simulink model "robocup_model"  (Simulink 8.6)
settings: Solver=ode45  StartTime=0.0  StopTime=8  RelTol=1e-3
libraries: fuzblock x3, simulink x3
settings Model: Creator=justbuchanan  LastModifiedBy=abdullah
settings SolverCC: ZeroCrossControl=EnableAll  ZeroCrossAlgorithm=Adaptive
settings DataIOCC: SignalLoggingSaveFormat=Dataset
settings OptimizationCC: BlockReduction=off  BufferReuse=off  ExpressionDepthLimit=128  SimCompilerOptimization=on
settings DebuggingCC: UnderspecifiedInitializationDetection=Simplified  MergeDetectMultiDrivingBlocksExec=error  FcnCallInpInsideContextMsg=EnableAllAsError  StateNameClashWarn=none
settings HardwareCC: ProdLargestAtomicInteger=Long  ProdLargestAtomicFloat=Double  ProdEndianess=LittleEndian  ProdHWDeviceType=ARM Compatible->ARM Cortex
settings GRTTargetCC: CombineOutputUpdateFcns=on  GRTInterface=off
settings ConfigComp: CovSFcnEnable=off

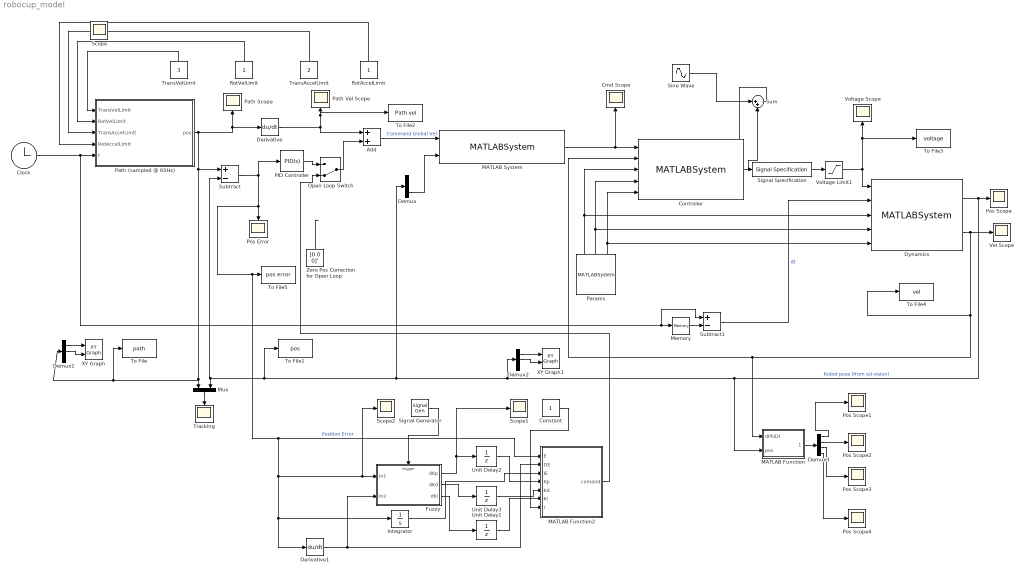
== system robocup_model ==
  Add : Sum
  Clock : Clock
  Cmd Scope : Scope
  Constant : Constant
  Controller : MATLABSystem  System=RobotLqr  trans_vel_weight=5  rot_vel_weight=0.1  u_weight=1  SimulateUsing=Interpreted execution
      mask Type: RobotLqr
      mask Display:
      | disp('RobotLqr');
      | port_label('input',1,'Cmd Velocity');
      | port_label('input',2,'Curr. Velocity');
      | port_label('input',3,'A_1');
      | port_label('input',4,'A_2');
      | port_label('input',5,'B');
      | port_label('output',1,'u');
  Demux : Demux  Outputs=3
  Demux1 : Demux  Outputs=3
  Demux2 : Demux  Outputs=3
  Demux3 : Demux
  Derivative : Derivative
  Derivative1 : Derivative
  Dynamics : MATLABSystem  System=Robot  SimulateUsing=Interpreted execution
      mask Type: Robot
      mask Display:
      | disp(['RoboCup Robot' char(10) 'Dynamics']);
      | port_label('input',1,'Motor Voltages');
      | port_label('input',2,'dt');
      | port_label('input',3,'A_1');
      | port_label('input',4,'A_2');
      | port_label('input',5,'B');
      | port_label('output',1,'Robot pose');
      | port_label('output',2,'Robot velocity');
  Fuzzy : Subsystem
  Integrator : Integrator
  MATLAB Function : MATLAB Function  TreatAsAtomicUnit=on
  MATLAB Function2 : MATLAB Function  TreatAsAtomicUnit=on
  MATLAB System : MATLABSystem  System=Global2Body  SimulateUsing=Code generation
      mask Type: Global2Body
      mask Display:
      | disp('Global2Body');
      | port_label('input',1,'Global Velocity');
      | port_label('input',2,'Robot angle');
      | port_label('output',1,'Body Velocity');
  Memory : Memory  X0=-0.1
  Mux : Mux  Inputs=2
  Open Loop Switch : ManualSwitch  CurrentSetting=0
  PID Controller : simulink/Continuous/PID Controller  Controller=PID  TimeDomain=Continuous-time  SampleTime=-1  IntegratorMethod=Forward Euler  FilterMethod=Forward Euler  Form=Parallel  UseFilter=on  ControllerParametersSource=internal  P=8  I=4  D=0  N=100  InitialConditionSource=internal  InitialConditionForIntegrator=0  InitialConditionForFilter=0  ExternalReset=none  LimitOutput=off  UpperSaturationLimit=inf  LowerSaturationLimit=-inf  LinearizeAsGain=on  AntiWindupMode=none  Kb=1  TrackingMode=off  Kt=1  PParamMin=[]  PParamMax=[]  IParamMin=[]  IParamMax=[]  DParamMin=[]  DParamMax=[]  NParamMin=[]  NParamMax=[]  KbParamMin=[]  KbParamMax=[]  KtParamMin=[]  KtParamMax=[]  POutMin=[]  POutMax=[]  IOutMin=[]  IOutMax=[]  DOutMin=[]  DOutMax=[]  NOutMin=[]  NOutMax=[]  KbOutMin=[]  KbOutMax=[]  KtOutMin=[]  KtOutMax=[]  IntegratorOutMin=[]  IntegratorOutMax=[]  FilterOutMin=[]  FilterOutMax=[]  SumOutMin=[]  SumOutMax=[]  SumI1OutMin=[]  SumI1OutMax=[]  SumI2OutMin=[]  SumI2OutMax=[]  SumI3OutMin=[]  SumI3OutMax=[]  SumDOutMin=[]  SumDOutMax=[]  SaturationOutMin=[]  SaturationOutMax=[]  IntegratorContinuousStateAttributes=''  IntegratorStateMustResolveToSignalObject=off  IntegratorRTWStateStorageClass=Auto  FilterContinuousStateAttributes=''  FilterStateMustResolveToSignalObject=off  FilterRTWStateStorageClass=Auto  DifferentiatorICPrevScaledInput=0  DifferentiatorOutMin=[]  DifferentiatorOutMax=[]
  Params : MATLABSystem  System=RobotParams  M_bot=2.205  I_bot=0.00745879949  g=2.0/7.0  r=0.0285623  L=0.0798576  Rt=0.464  K_e=30.0/(380*pi)  K_t=0.0251  K_f=0.0001  I_asm=2.43695253e-5  V=18  wheel_angles=[38*pi/180.0, 142*pi/180.0, 225*pi/180.0, 315*pi/180.0]'  SimulateUsing=Code generation
      mask Type: RobotParams
      mask Display:
      | disp('RobotParams');
      | port_label('output',1,'A_1');
      | port_label('output',2,'A_2');
      | port_label('output',3,'B');
  Path (sampled @ 60Hz) : MATLAB Function  TreatAsAtomicUnit=on  SystemSampleTime=1/60
  Path Scope : Scope
  Path Vel Scope : Scope
  Pos Error : Scope
  Pos Scope{,1..4} (5 alike) : Scope
  RotAccelLimit : Constant
  RotVelLimit : Constant
  Scope1 : Scope
  Scope2 : Scope
  Signal Generator : SignalGenerator  WaveForm=square  Frequency=0.05  Units=rad/sec
  Signal Specification : SignalSpecification  OutDataTypeStr=double  Dimensions=[4 1]
  Sine Wave : Sin  Amplitude=0  SampleTime=0
  Subtract : Sum  Inputs=+-
  Subtract1 : Sum  Inputs=+-
  Sum : Sum  Inputs=|++
  To File : ToFile  Filename=path  MatrixName=path_pir
  To File1 : ToFile  Filename=pos  MatrixName=pos_pir
  To File2 : ToFile  Filename=Path vel  MatrixName=path_vel_pir
  To File3 : ToFile  Filename=voltage  MatrixName=voltage_pir
  To File4 : ToFile  Filename=vel  MatrixName=vel_pir
  To File5 : ToFile  Filename=pos error  MatrixName=pos_error_pir
  Tracking : Scope
  TransAccelLimit : Constant  Value=2
  TransVelLimit : Constant  Value=3
  Unit Delay1 : UnitDelay  InitialCondition=[0 0 0]  SampleTime=0.5
  Unit Delay2 : UnitDelay  InitialCondition=[0 0 0]  SampleTime=0.5
  Unit Delay3 : UnitDelay  InitialCondition=[0 0 0]  SampleTime=0.5
  Vel Scope : Scope
  Voltage Limit1 : Saturate  UpperLimit=18  LowerLimit=-18
  Voltage Scope : Scope
  XY Graph : simulink/Sinks/XY Graph  xmin=-1  xmax=2.5  ymin=-1  ymax=2.5  st=-1
  XY Graph1 : simulink/Sinks/XY Graph  xmin=-1  xmax=2.5  ymin=-1  ymax=2.5  st=-1
  Zero Pos Correction for Open Loop : Constant  Value=[0 0 0]'
  Scope : Scope
  wires:
  Derivative/1 -> Add/1, To File2/1, Path Vel Scope/1
  Path (sampled @ 60Hz)/1(pos) -> Derivative/1, Path Scope/1, Subtract/1, Demux1/1, To File/1, Mux/1
  Add/1 -> MATLAB System/1  "Command Global Vel"
  Subtract1/1 -> Dynamics/2  "dt"
  Params/1 -> Controller/3, Dynamics/3
  Params/2 -> Controller/4, Dynamics/4
  Params/3 -> Controller/5, Dynamics/5
  Dynamics/1 -> MATLAB Function/2(pos), Demux2/1, Demux/1, To File1/1, Subtract/2, Mux/2, Pos Scope/1  "Robot pose (from ssl-vision)"
  Dynamics/2 -> Vel Scope/1, MATLAB Function/1(dPhiDt), Controller/2, To File4/1
  TransVelLimit/1 -> Path (sampled @ 60Hz)/1(TransVelLimit)
  RotVelLimit/1 -> Path (sampled @ 60Hz)/2(RotVelLimit)
  TransAccelLimit/1 -> Path (sampled @ 60Hz)/3(TransAccelLimit)
  RotAccelLimit/1 -> Path (sampled @ 60Hz)/4(RotAccelLimit)
  Clock/1 -> Subtract1/1, Memory/1, Path (sampled @ 60Hz)/5(t)
  Memory/1 -> Subtract1/2
  Open Loop Switch/1 -> Add/2
  Zero Pos Correction for Open Loop/1 -> ?
  Mux/1 -> Tracking/1
  Signal Specification/1 -> Voltage Limit1/1
  MATLAB System/1 -> Controller/1, Cmd Scope/1
  Demux/3 -> MATLAB System/2
  Demux1/1 -> XY Graph/1
  Demux1/2 -> XY Graph/2
  Demux2/1 -> XY Graph1/1
  Demux2/2 -> XY Graph1/2
  Sine Wave/1 -> Sum/1
  Controller/1 -> Sum/2
  Sum/1 -> Signal Specification/1
  PID Controller/1 -> Open Loop Switch/1
  Subtract/1 -> PID Controller/1, MATLAB Function2/1(E), Scope2/1, Fuzzy/1(In1), Derivative1/1, Integrator/1, To File5/1, Pos Error/1  "Position Error"
  Derivative1/1 -> MATLAB Function2/2(DE), Fuzzy/2(In2)
  Fuzzy/1(dKp) -> Scope1/1, Unit Delay2/1
  Fuzzy/2(dKd) -> Unit Delay3/1
  Unit Delay2/1 -> MATLAB Function2/4(Kp)
  Unit Delay3/1 -> MATLAB Function2/5(Kd)
  MATLAB Function2/1(comand) -> Open Loop Switch/2
  Signal Generator/1 -> Fuzzy/Trigger
  Fuzzy/3(dKi) -> Unit Delay1/1
  Unit Delay1/1 -> MATLAB Function2/6(Ki)
  Integrator/1 -> MATLAB Function2/3(IE)
  Constant/1 -> MATLAB Function2/7(r)
  Voltage Limit1/1 -> To File3/1, Voltage Scope/1, Dynamics/1
  MATLAB Function/1(wheels) -> Demux3/1
  Demux3/1 -> Pos Scope1/1
  Demux3/2 -> Pos Scope2/1
  Demux3/3 -> Pos Scope3/1
  Demux3/4 -> Pos Scope4/1

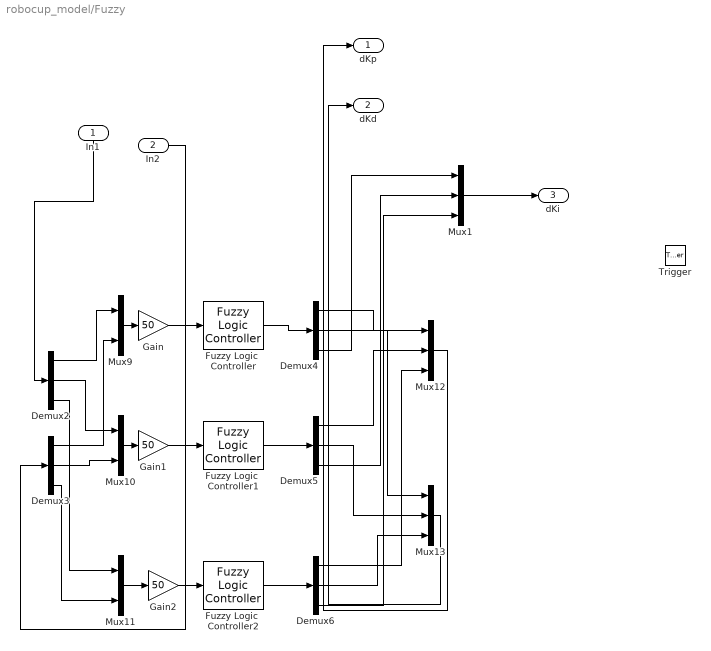
== system robocup_model/Fuzzy ==
  In1 : Inport
  In2 : Inport  Port=2
  Trigger : TriggerPort  PortDimensions=1
  Demux{2..6} (5 alike) : Demux  Outputs=3
  Fuzzy Logic  Controller : fuzblock/Fuzzy Logic  Controller  fis=readfis('C3.fis')
  Fuzzy Logic  Controller1 : fuzblock/Fuzzy Logic  Controller  fis=readfis('C3.fis')
  Fuzzy Logic  Controller2 : fuzblock/Fuzzy Logic  Controller  fis=readfis('C3.fis')
  Gain : Gain  Gain=50
  Gain1 : Gain  Gain=50
  Gain2 : Gain  Gain=50
  Mux1 : Mux  Inputs=3
  Mux10 : Mux  Inputs=2
  Mux11 : Mux  Inputs=2
  Mux12 : Mux  Inputs=3
  Mux13 : Mux  Inputs=3
  Mux9 : Mux  Inputs=2
  dKp : Outport
  dKd : Outport  Port=2
  dKi : Outport  Port=3
  wires:
  Mux11/1 -> Gain2/1
  Demux3/1 -> Mux9/2
  Demux3/3 -> Mux11/2
  Demux2/2 -> Mux10/1
  Demux2/1 -> Mux9/1
  Demux2/3 -> Mux11/1
  Mux13/1 -> dKd/1
  Mux12/1 -> dKp/1
  Demux4/2 -> Mux13/1
  Demux5/2 -> Mux13/2
  Demux6/1 -> Mux12/3
  Mux9/1 -> Gain/1
  Demux5/1 -> Mux12/2
  Mux10/1 -> Gain1/1
  Demux6/2 -> Mux13/3
  Fuzzy Logic  Controller1/1 -> Demux5/1
  Fuzzy Logic  Controller2/1 -> Demux6/1
  Fuzzy Logic  Controller/1 -> Demux4/1
  In2/1 -> Demux3/1
  Demux4/1 -> Mux12/1
  In1/1 -> Demux2/1
  Demux3/2 -> Mux10/2
  Mux1/1 -> dKi/1
  Demux4/3 -> Mux1/1
  Demux5/3 -> Mux1/2
  Demux6/3 -> Mux1/3
  Gain/1 -> Fuzzy Logic  Controller/1
  Gain1/1 -> Fuzzy Logic  Controller1/1
  Gain2/1 -> Fuzzy Logic  Controller2/1

== matlab function MATLAB Function ==
  data: dPhiDt input double; wheels output double; pos input double
function wheels = fcn(dPhiDt,pos)
phi=pos(3);
gbR = [cos(phi), -sin(phi), 0;
           sin(phi),  cos(phi), 0;
                  0,         0, 1];


D = [-sin(-45*pi/180) cos(-45*pi/180) 1
     -sin(45*pi/180) cos(45*pi/180) 1
     -sin(135*pi/180) cos(135*pi/180) 1
     -sin(-135*pi/180) cos(-135*pi/180) 1];
    wheels = D*inv(gbR)*dPhiDt;

== matlab function Path (sampled @ 60Hz) ==
  data: TransVelLimit input double; RotVelLimit input double; TransAccelLimit input double; RotAccelLimit input double; pos output double; t input double
function pos = path(TransVelLimit, RotVelLimit, TransAccelLimit, RotAccelLimit, t)
%#codegen

pos = [0 0 0]';

accel = [1 0 0.01]';


% rampTime = TransVelLimit/TransAccelLimit;
% flatTime = 2;
% % 
% % 
% % ramp-up
% pos = pos + 0.5*accel*min(t,rampTime)^2;
% 
% % const speed
% if t > rampTime
%     vel = accel*rampTime;
%     pos = pos + min(t-rampTime, flatTime)*vel;
% end
% 
% % ramp-down
% if t > rampTime + flatTime
%     vi = accel*rampTime;
%     rampDownT = min(t-rampTime-flatTime, rampTime);
%     pos = pos + -0.5*accel*rampDownT^2 + vi*rampDownT;
% end


% circular path
% pos = [sin(t*.8) cos(t*.8) 0]';

% Rectangular path t=4
% if t < 1 && t > 0
%     pos = [t,0,0]';
% end
% if t < 2 && t>= 1
%     pos = [1,t-1,0]';
% end
% if t < 3 && t>= 2
%     pos = [1-(t-2),1,0]';
% end
% if t < 4 && t>= 3
%     pos = [0,1-(t-3),0]';
% end

% Rectangular path t=8
% if t < 2 && t > 0
%     pos = [t,0,0]';
% end
% if t < 4 && t>= 2
%     pos = [2,t-2,0]';
% end
% if t < 6 && t>= 4
%     pos = [2-(t-4),2,0]';
% end
% if t < 8 && t>= 6
%     pos = [0,2-(t-6),0]';
% end


%%
x=5*0.1*sin(3*t);
y=5*0.3*cos(1*t);
pos=[x,y,0]';
% t=0:60;
% t = linspace(0, 2*pi, 360);
% x=sin(t);
% y=cos(t);
% plot(x)
% plot(y)
% plot(x,y)

== matlab function MATLAB Function2 ==
  data: E input double; DE input double; IE input double; Kp input double; Kd input double; comand output double; Ki input double; r input double
function comand  = fcn(E,DE,IE,Kp,Kd,Ki,r)
comand=zeros(3,1);
Kp=Kp*r;
Kd=Kd*r;
Ki=Ki*r;
comand(1)=E(1)*(8*Kp(1)+8)+IE(1)*(4*Ki(1)+4);
comand(2)=E(2)*(8*Kp(2)+8)+IE(2)*(4*Ki(2)+4);
comand(3)=E(3)*(8*Kp(3)+8)+IE(3)*(4*Ki(3)+4);

% comand(3)=E(3)*(4*Kp(3)+8)+IE(3)*(0.5*Ki(3)+4)+DE(3)*(0.5*Kd(3)+0);
